simulink model "model"  (R2020b)
settings: Solver=VariableStepAuto  StartTime=0.0  StopTime=50  RelTol=1e-3
settings Model: Creator=Vrunda M Balgi  LastModifiedBy=Avengers

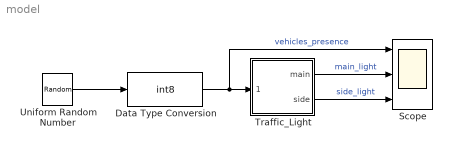
== system model ==
  Data Type Conversion : DataTypeConversion  OutDataTypeStr=int8  RndMeth=Nearest
  Scope : Scope  NumInputPorts=3
  Traffic_Light : Stateflow chart  TreatAsAtomicUnit=on
  Uniform Random Number : UniformRandomNumber  Minimum=0  SampleTime=0.25
  wires:
  Uniform Random Number/1 -> Data Type Conversion/1
  Data Type Conversion/1 -> Scope/1, Traffic_Light/1(vehicle)  "vehicles_presence"
  Traffic_Light/1(main) -> Scope/2  "main_light"
  Traffic_Light/2(side) -> Scope/3  "side_light"

== stateflow chart model/Traffic_Light ==
  settings: stateMachineType=MOORE_MACHINE
  state FirstState
    main = GREEN;
    side = RED;
  state SecondState
    main = YELLOW;
    side = RED;
  state ThirdState
    main = RED;
    side = RED;
  state SixthState
    main = RED;
    side = RED;
  state FifthState
    main = RED;
    side = YELLOW;
  state FourthState
    main = RED;
    side = GREEN;
  (default) -> FirstState
  FirstState -> SecondState : [vehicle==1 || after(25,tick)]
  SecondState -> ThirdState : after(4,tick)
  SixthState -> FirstState : after(1,tick)
  ThirdState -> FourthState : after(1,tick)
  FifthState -> SixthState : after(4,tick)
  FourthState -> FifthState : [vehicle==0 && after(25,tick)]
  data: GREEN constant double =3; YELLOW constant double =2; RED constant double =1; main output; side output; vehicle input
